simulink model "effeciency"  (R2024a)
settings: Solver=ode45  StartTime=0.0  StopTime=0.1  MaxStep=500000  RelTol=1e-3
libraries: spsPowerLib x2, spsRMSLib x2, spsCurrentMeasurementLib x2, spsVoltageMeasurementLib x2, spsACVoltageSourceLib x1, spsLinearTransformerLib x1, spsSeriesRLCBranchLib x1, sps_lib x1
settings Model: Creator=Jagan mohan  LastModifiedBy=Jagan mohan
settings DataIOCC: MaxDataPoints=500000  SaveFinalState=on  SaveState=on  InspectSignalLogs=on  LoggingToFile=on

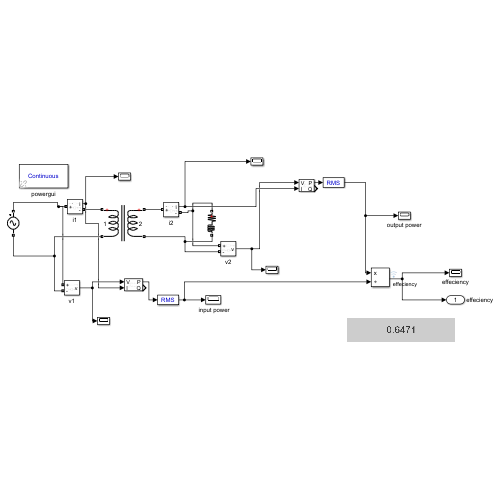
[thumbnail: Simulink's stored preview of the top-level diagram]
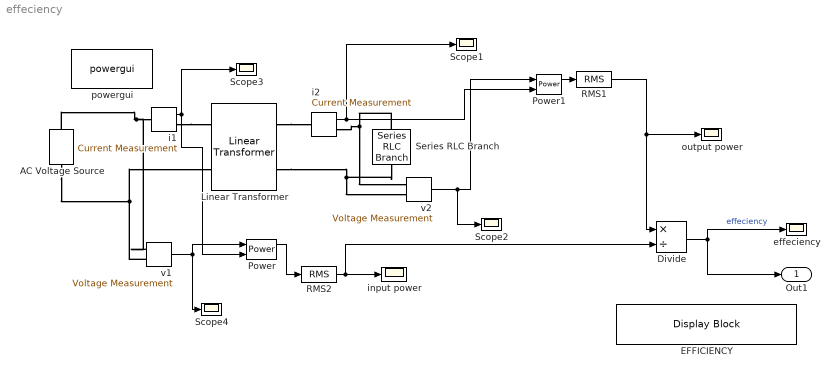
== system effeciency ==
  " input power" : Scope
  AC Voltage Source : spsACVoltageSourceLib/AC Voltage Source  Amplitude=220  Phase=0  Frequency=60  SampleTime=0  Measurements=None  BusType=swing  Pref=10e3  Qref=0  Qmin=-inf  Qmax=+inf
  Divide : Product  Inputs=*/
  EFFICIENCY : DisplayBlock  LabelPosition=Hide  Transparency=1
  Linear Transformer : spsLinearTransformerLib/Linear Transformer  UNITS=SI  NominalPower=[ 250e6 60 ]  winding1=[155.586 4 0.4]  winding2=[311.174 0.8 0.08]  ThreeWindings=off  winding3=[3.15e+05 0.7938 0.084225]  RmLm=[1000 2]  Measurements=None  DataType=on
  Power : spsPowerLib/Power  Freq=60  Vinit=[1, 0]  Iinit=[1, 0]  Ts=0
  Power1 : spsPowerLib/Power  Freq=60  Vinit=[1, 0]  Iinit=[1, 0]  Ts=0
  RMS1 : spsRMSLib/RMS  TrueRMS=on  Freq=50  RMSInit=0  Ts=0
  RMS2 : spsRMSLib/RMS  TrueRMS=on  Freq=50  RMSInit=0  Ts=0
  Scope{1..4} (4 alike) : Scope
  Series RLC Branch : spsSeriesRLCBranchLib/Series RLC Branch  LConnTagsString=__new0  RConnTagsString=__new0  BranchType=RL  Resistance=1000  Inductance=1  SetiL0=off  InitialCurrent=0  Capacitance=1e-6  Setx0=off  InitialVoltage=0  Measurements=None
  effeciency : Scope
  i1 : spsCurrentMeasurementLib/Current Measurement  PhasorSimulation=off  OutputType=Complex  PSBequivalent=0
  i2 : spsCurrentMeasurementLib/Current Measurement  PhasorSimulation=off  OutputType=Complex  PSBequivalent=0
  output power : Scope
  powergui : sps_lib/powergui  Priority=1  SimulationMode=Continuous  SampleTime=5  frequency=60  Iterations=50  frequencyindice=60  Pbase=100e6  ErrMax=1e-4  UnitsV=kV  UnitsW=MW  buscounter=0  FunctionMessages=off  echomessages=off  EnableUseOfTLC=off  CurrentSourceSwitches=off  DisableSnubberDevices=off  DisableRonSwitches=off  DisableVfSwitches=off  DisplayEquations=off  AutomaticDiscreteSolvers=off  SolverType=Tustin/Backward Euler (TBE)  Interpol=off  ExternalGateDelay=off  methode=off  Ts=100  x0status=blocks  SPID=on  SwTol=0  HookPort=off  NonlinearTolerance=1e-4  nMaxIteration=100  ContinueOnMaxIteration=off  RestoreLinks=warning  ResistiveCurrentMeasurement=off  Frange=[0:2:500]  Ylog=off  Xlog=on  ShowGrid=off  save=off  variable=ZData  structure=0  ZoomFFT=off  StartTime=0.0  cycles=1  DisplayStyle=1  fundamental=60  FreqAxis=off  MaxFrequency=1000  frequencyindicesteady=1  RmsSteady=1  display=off
  v1 : spsVoltageMeasurementLib/Voltage Measurement  PhasorSimulation=off  OutputType=Complex  PSBequivalent=0
  v2 : spsVoltageMeasurementLib/Voltage Measurement  PhasorSimulation=off  OutputType=Complex  PSBequivalent=0
  Out1 : Outport  SignalName=effeciency
  wires:
  v1/1 -> Power/1, Scope4/1
  i1/1 -> Power/2, Scope3/1
  v2/1 -> Scope2/1, Power1/1
  i2/1 -> Scope1/1, Power1/2
  Power/1 -> RMS2/1
  RMS2/1 -> Divide/2, " input power"/1
  Power1/1 -> RMS1/1
  RMS1/1 -> Divide/1, output power/1
  Divide/1 -> Out1/1, effeciency/1  "effeciency"
  connections:
  Linear Transformer/RConn2 -- v2/LConn2 -- Series RLC Branch/RConn1
  AC Voltage Source/LConn1 -- Linear Transformer/LConn2 -- v1/LConn2
  i1/RConn1 -- Linear Transformer/LConn1
  AC Voltage Source/RConn1 -- v1/LConn1 -- i1/LConn1
  Linear Transformer/RConn1 -- i2/LConn1
  i2/RConn1 -- v2/LConn1 -- Series RLC Branch/LConn1
